simulink model "sdrrTVWhiteSpaceMonitorRPiExample"  (R2020b)
settings: Solver=FixedStepDiscrete  StartTime=0.0  StopTime=inf  RelTol=1e-3  EnableMultiTasking=on
libraries: sdrrblksprivate x1, sdrrlib x1, dspspect3 x1
settings Model: SimulationMode=external  ExtModeTrigDuration=100  Creator=The MathWorks, Inc.  LastModifiedBy=The MathWorks, Inc.
settings SolverCC: PositivePriorityOrder=on
settings DataIOCC: LimitDataPoints=on  SaveFormat=Array  SaveOutput=off  SignalLogging=off  DSMLogging=off  SaveTime=off  ReturnWorkspaceOutputs=off
settings OptimizationCC: PassReuseOutputArgsThreshold=0  ExpressionDepthLimit=2147483647  MaxStackSize=64
settings DebuggingCC: UnderspecifiedInitializationDetection=Classic  MergeDetectMultiDrivingBlocksExec=none  ParameterPrecisionLossMsg=none  ParameterTunabilityLossMsg=error  FcnCallInpInsideContextMsg=warning  AllowSymbolicDim=off  StateNameClashWarn=warning  SFUnexpectedBacktrackingDiag=warning  SFNoUnconditionalDefaultTransitionDiag=warning  SFExecutionAtInitializationDiag=none  ArithmeticOperatorsInVariantConditions=warning
settings HardwareCC: ProdBitPerPointer=32  ProdBitPerSizeT=32  ProdBitPerPtrDiffT=32  ProdLargestAtomicInteger=Long  ProdLargestAtomicFloat=Double  ProdWordSize=32  ProdHWDeviceType=ARM Compatible->ARM Cortex  TargetBitPerLong=64  TargetBitPerPointer=64  TargetBitPerSizeT=64  TargetBitPerPtrDiffT=64  TargetLongLongMode=on  TargetIntDivRoundTo=Zero  TargetEndianess=LittleEndian  TargetWordSize=64  TargetHWDeviceType=Generic->MATLAB Host Computer  UseEmbeddedCoderFeatures=off
settings ModelReferenceCC: PropagateSignalLabelsOutOfModel=off
settings SFSimCC: SimUseLocalCustomCode=off  MATLABDynamicMemAlloc=off  CustomCodeUndefinedFunction=UseInterfaceOnly
settings RTWCC: Description=Embedded Coder  SystemTargetFile=ert.tlc  HardwareBoard=Raspberry Pi  TLCOptions="-aInlineSetEventsForThisBaseRateFcn=TLC_FALSE -aSuppressMultiTaskScheduler=TLC_FALSE  -aRateBasedStepFcn=0"  TemplateMakefile=ert_default_tmf  GenerateReport=on  RTWVerbose=off  RTWUseLocalCustomCode=off  Toolchain=GNU GCC Raspberry Pi  BuildConfiguration=Faster Runs  LaunchReport=on
settings RTWCC: CustomSourceCode=|
  | #include<stdio.h>
  | #include<stdlib.h>
settings CodeAppCC: ForceParamTrailComments=on  OperatorAnnotations=on
settings ERTTargetCC: ERTCustomFileBanners=off  SupportContinuousTime=on  SupportNonInlinedSFcns=on  RemoveResetFunc=off  SupportVariableSizeSignals=on  ModelStepFunctionPrototypeControlCompliant=off
settings ConfigComp: CovMetricSettings=dw  CovSaveCumulativeToWorkspaceVar=on  CovSaveSingleToWorkspaceVar=on  CovExternalEMLEnable=off  CovSFcnEnable=off

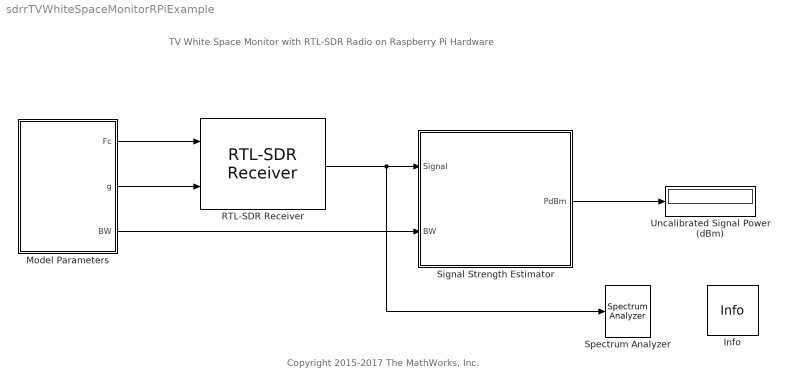
== system sdrrTVWhiteSpaceMonitorRPiExample ==
  note: TV White Space Monitor with RTL-SDR Radio
      | on Raspberry Pi Hardware
  note: Copyright 2015-2017 The MathWorks, Inc.
  Info : sdrrblksprivate/Info  SystemSampleTime=-1  VariantActivationTime=update diagram  Latency=0  AutoFrameSizeCalculation=off
  Model Parameters : Subsystem  mask(Model Parameters){fc=561.25, bw2=200, gain=50}
      mask prompts: fc "Center frequency (MHz):"; bw2 "Two-sided bandwidth (kHz):"; gain "Gain (dB):"
      mask help:
      | Choose TV white space monitor parameters.
      |
      | You can select center frequency of the band you want to monitor. You can set the two-sided bandwidth, which must be less than 2400 kHz. You can also set the tuner gain of the RTL-SDR radio.
      settings: AttributesFormatString=|
      | Fc: %<fc> MHz
      | BW: %<bw2> kHz
      | Gain: %<gain> dB
      mask Help: eval('sdrrdemohelp');
      mask Callback fc:
      | paramBlock = gcb;
      | fc = eval(get_param(paramBlock, 'fc'));
      | set_param([paramBlock '/Center Frequency'], 'Value', num2str(fc*1e6));
      | scope = get_param([bdroot '/Spectrum Analyzer'], 'ScopeConfiguration');
      | scope.FrequencyOffset = num2str(fc*1e6);
      | clear paramBlock fc scope
      mask Callback bw2:
      | paramBlock = gcb;
      | bw2 = eval(get_param(paramBlock, 'bw2'));
      | set_param([paramBlock '/Two-sided BW'], 'Value', num2str(bw2*1e3));
      | clear paramBlock bw2
      mask Callback gain:
      | paramBlock = gcb;
      | gain = get_param(gcb, 'gain');
      | set_param([paramBlock '/Gain'], 'Value', gain);
      | clear paramBlock gain
      mask Display: disp('Model\nParameters')
  RTL-SDR Receiver : sdrrlib/RTL-SDR Receiver  IPAddress=0  CenterFrequencySource=Input port  CenterFrequency=102.5e6  GainSource=Input port  Gain=50  ADCRate=2.4e6  FrequencyCorrection=0  LostSamplesOutputPort=off  LatencyOutputPort=off  OutputDataType=double  FrameLength=256*20  EnableBurstMode=off  NumFramesInBurst=20  sobjType=sdrr.internal.SDRRTLReceiverSL  dataUDPPort=-1  ctrlUDPPort=-1  subDeviceList=nosubdev  sdrBlockType=SDRBlockTypeSLT.SDRRxBlock  requester=UNUSED_BY_SFCN  sdrExecutionMode=SDRExecutionModeSLT.ExecModeHW  BypassUserLogic=off  DecimatorSelect=DDC decimator  SourceSelect=Sine generator  SineAmplitude=16000  EnableInternalClock=off  BypassIQBalance=off  IFBandwidth=40e6  ADCRateSource=Dialog  IntermediateFrequency=0  DecimationFactorSource=Dialog  DecimationFactor=512  RFFrequencyIsTunable=logical(1)  SampleTime=(256*20)/(2.4e6)  IFBandwidthSource=Dialog  SineFrequency=30000  BypassDCBlockingFilter=off  IntermediateFrequencySource=Dialog  IQBalanceCoefficients=64  SkipAllHardwareResetAndInitialization=off  EnableIQCalibrationTable=on  CacheIQCalibrationTable=off  EnableOffsetTuning=off  EnableRTLAGC=off  EnableTestMode=off  EnableTunerAGC=off  FrequencyCorrectionSource=Dialog  NumMLBuffers=128  NumUSBBuffers=16  RTLCrystalFrequency=28800000  TunerCrystalFrequency=28800000
      settings: SourceProductName=Communications Toolbox Support Package for RTL-SDR Radio
  Signal Strength Estimator : Subsystem
  Spectrum Analyzer : SpectrumAnalyzer
  Uncalibrated Signal Power (dBm) : Display
  wires:
  Model Parameters/2(g) -> RTL-SDR Receiver/2
  Model Parameters/1(Fc) -> RTL-SDR Receiver/1
  RTL-SDR Receiver/1 -> Spectrum Analyzer/1, Signal Strength Estimator/1(Signal)
  Signal Strength Estimator/1(PdBm) -> Uncalibrated Signal Power (dBm)/1
  Model Parameters/3(BW) -> Signal Strength Estimator/2(BW)

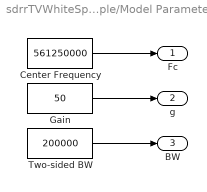
== system sdrrTVWhiteSpaceMonitorRPiExample/Model Parameters ==
  Center Frequency : Constant  Value=561250000
  Gain : Constant  Value=50
  Two-sided BW : Constant  Value=200000
  Fc : Outport  VectorParamsAs1DForOutWhenUnconnected=off
  g : Outport  Port=2  VectorParamsAs1DForOutWhenUnconnected=off
  BW : Outport  Port=3  VectorParamsAs1DForOutWhenUnconnected=off
  wires:
  Gain/1 -> g/1
  Center Frequency/1 -> Fc/1
  Two-sided BW/1 -> BW/1

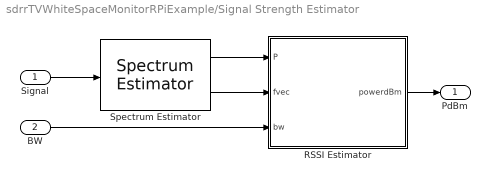
== system sdrrTVWhiteSpaceMonitorRPiExample/Signal Strength Estimator ==
  Signal : Inport
  BW : Inport  Port=2
  RSSI Estimator : MATLAB Function  TreatAsAtomicUnit=on
  Spectrum Estimator : dspspect3/Spectrum Estimator  Method=Welch  NumTapsPerBand=12  SpectrumType=Power  FrequencyResolutionMethod=Window length  FilterBankResolutionMethod=Number of frequency bands  RBW=5  WindowLength=1024  FrequencyBandsSource=Same as input frame size  FrequencyBands=1024  FFTLengthSource=Property  FFTLength=2^14  InheritSampleRate=on  SampleRate=44100  Window=Hann  SidelobeAttenuation=60  AveragingMethod=Running  SpectralAverages=1  ForgettingFactorPort=off  ForgettingFactor=0.9  Overlap=0  ReferenceLoad=1  FrequencyRange=Centered  PowerUnits=Watts  OutputMaxHoldSpectrum=off  OutputMinHoldSpectrum=off  OutputFrequencyVector=on  OutputRBW=off  SimulateUsing=Code generation
      settings: SourceProductName=DSP System Toolbox
  PdBm : Outport  VectorParamsAs1DForOutWhenUnconnected=off
  wires:
  BW/1 -> RSSI Estimator/3(bw)
  RSSI Estimator/1(powerdBm) -> PdBm/1
  Signal/1 -> Spectrum Estimator/1
  Spectrum Estimator/1 -> RSSI Estimator/1(P)
  Spectrum Estimator/2 -> RSSI Estimator/2(fvec)

== matlab function sdrrTVWhiteSpaceMonitorRPiExample/Signal Strength Estimator/RSSI Estimator ==
  data: P input; powerdBm output; fvec input [0..3.2e6]; bw input
function powerdBm = rssi(P, fvec, bw)
%#codegen

powerWatt = sum(P(abs(fvec) < bw/2));
powerdBm = 10*log10(powerWatt/1e-3);
